simulink model "aeroplt2"  (Simulink 5.0)
settings: Solver=ode1  StartTime=0.0  StopTime=t_in(end)  FixedStep=.02  RelTol=1e-3
values from neighbouring files (symbols this model uses):
  b = 124.524    [gp.m]    (also in trim_541.mat)
  Cbar = 16.64    [gp.m]    (also in trim_541.mat)
  CG = 0.25    [gp.m]    (also in trim_541.mat)
  cs = 1100    [gp.m]    (also in trim_541.mat = 1097.09545231)
  EAS = 210    [gp.m]    (also in trim_541.mat = 209.982128693)
  QBAR = 150    [gp.m]    (also in trim_541.mat = 149.275292764)
  RunwayAlt = 9    [gp.m]    (also in trim_541.mat)
  S = 1951    [gp.m]    (also in trim_541.mat)
  splr_vec = 0:splr_step:10    [gp.m]    (also in gp.mat = [0 2 4 6 8 10])
  StatesInp = [380.111621264 0 35.7647907785 0 -1.82640716025e-05 0 5000 0.698131700798 -1.29154364648 0 0.0938140386005 0 ... (15 elements, 15x1)]    [trim_541.mat]
  weight = 185000    [gp.m]    (also in trim_541.mat)
libraries: simulink x4
settings Model: Creator=wtb  LastModifiedBy=Gpapageo  ExtModeAutoUpdateStatusClock=off  BooleanDataType=off

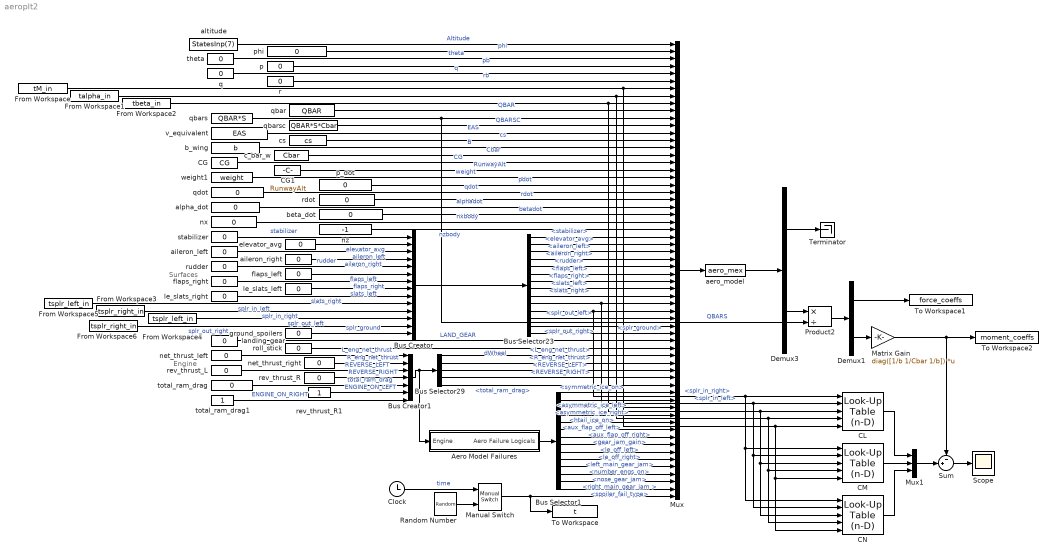
== system aeroplt2 ==
  note: Surfaces
  note: Engine
  " aileron_right" : Constant  Value=0
  Aero Model Failures : Subsystem
  Bus Creator : BusCreator  Inputs=14
  Bus Creator1 : BusCreator  Inputs=7
  Bus Selector1 : BusSelector  OutputSignals=symmetric_ice_on,asymmetric_ice_left,asymmetric_ice_right,htail_ice_on,aux_flap_off_left,aux_flap_off_right,gear_jam_gain,le_off_left,le_off_right,left_main_gear_jam,number_engs_on,nose_gear_jam,right_main_gear_jam ,spoiler_fail_type
  Bus Selector23 : BusSelector  OutputSignals=stabilizer,elevator_avg,aileron_left,aileron_right,rudder,flaps_left,flaps_right,slats_left,slats_right,splr_in_left,splr_in_right,splr_out_left,splr_out_right,splr_ground
  Bus Selector29 : BusSelector  OutputSignals=L_eng_net_thrust,R_eng_net_thrust,REVERSE_LEFT,REVERSE_RIGHT,total_ram_drag
  CG : Constant  Value=CG
  CG1 : Constant  Value=RunwayAlt
  CL : simulink/Look-Up Tables/Look-Up Table (n-D)  numDimsPopupSelect=More...  bp1=splr_vec  bp2=splr_vec  bp3=beta_vec  bp4=alpha_vec  bpcell={M_vec}  explicitNumDims=5  searchMode=Binary Search  cacheBpFlag=on  vectorInputFlag=off  tableData=CL_mat  interpMethod=Linear  extrapMethod=Linear  rangeErrorMode=None
  CM : simulink/Look-Up Tables/Look-Up Table (n-D)  numDimsPopupSelect=More...  bp1=splr_vec  bp2=splr_vec  bp3=beta_vec  bp4=alpha_vec  bpcell={M_vec}  explicitNumDims=5  searchMode=Binary Search  cacheBpFlag=on  vectorInputFlag=off  tableData=CM_mat  interpMethod=Linear  extrapMethod=Linear  rangeErrorMode=None
  CN : simulink/Look-Up Tables/Look-Up Table (n-D)  numDimsPopupSelect=More...  bp1=splr_vec  bp2=splr_vec  bp3=beta_vec  bp4=alpha_vec  bpcell={M_vec}  explicitNumDims=5  searchMode=Binary Search  cacheBpFlag=on  vectorInputFlag=off  tableData=CN_mat  interpMethod=Linear  extrapMethod=Linear  rangeErrorMode=None
  Clock : Clock
      settings: Decimation=10
  Demux1 : Demux  Outputs=[3 3]
  Demux3 : Demux  Outputs=[7 6]
  From Workspace : FromWorkspace  VariableName=tM_in  SampleTime=.02
  From Workspace1 : FromWorkspace  VariableName=talpha_in  SampleTime=.02
  From Workspace2 : FromWorkspace  VariableName=tbeta_in  SampleTime=.02
  From Workspace3 : FromWorkspace  VariableName=tsplr_right_in  SampleTime=.02
  From Workspace4 : FromWorkspace  VariableName=tsplr_left_in  SampleTime=.02
  From Workspace5 : FromWorkspace  VariableName=tsplr_left_in  SampleTime=.02
  From Workspace6 : FromWorkspace  VariableName=tsplr_right_in  SampleTime=.02
  Manual Switch : simulink/Signal Routing/Manual Switch  sw=1  action=0
  Matrix Gain : Gain  Gain=diag([1/b 1/Cbar 1/b])  Multiplication=Matrix(K*u)  SaturateOnIntegerOverflow=on
  Mux : Mux  Inputs=62
  Mux1 : Mux  Inputs=3
  Product2 : Product  Inputs=*/  SaturateOnIntegerOverflow=on
  Random Number : RandomNumber  SampleTime=0
  Scope : Scope
      settings: YMin=-3.5e-018  YMax=3.5e-018
  Sum : Sum  Inputs=-+|  SaturateOnIntegerOverflow=on
  Terminator : Terminator
  To Workspace : ToWorkspace  VariableName=t  SampleTime=.02  SaveFormat=Array
  To Workspace1 : ToWorkspace  VariableName=force_coeffs  SampleTime=-1  SaveFormat=Array
  To Workspace2 : ToWorkspace  VariableName=moment_coeffs  SampleTime=-1  SaveFormat=Array
  aero_model : S-Function  FunctionName=aero_mex
  aileron_left : Constant  Value=0
  alpha_dot : Constant  Value=0
  altitude : Constant  Value=StatesInp(7)
  b_wing : Constant  Value=b
  beta_dot : Constant  Value=0
  c_bar_w : Constant  Value=Cbar
  cs : Constant  Value=cs
  elevator_avg : Constant  Value=0
  flaps_left : Constant  Value=0
  flaps_right : Constant  Value=0
  ground_spoilers : Constant  Value=0
  landing_gear : Constant  Value=0
  le_slats_left : Constant  Value=0
  le_slats_right : Constant  Value=0
  net_thrust_left : Constant  Value=0
  net_thrust_right : Constant  Value=0
  nx : Constant  Value=0
  nz : Constant  Value=-1
  p : Constant  Value=0
  p_dot : Constant  Value=0
  phi : Constant  Value=0
  q : Constant  Value=0
  qbar : Constant  Value=QBAR
  qbars : Constant  Value=QBAR*S
  qbarsc : Constant  Value=QBAR*S*Cbar
  qdot : Constant  Value=0
  r : Constant  Value=0
  rdot : Constant  Value=0
  rev_thrust_L : Constant  Value=0
  rev_thrust_R : Constant  Value=0
  rev_thrust_R1 : Constant
  roll_stick : Constant  Value=0
  rudder : Constant  Value=0
  stabilizer : Constant  Value=0
  theta : Constant  Value=0
  total_ram_drag : Constant  Value=0
  total_ram_drag1 : Constant
  v_equivalent : Constant  Value=EAS
  weight1 : Constant  Value=weight
  wires:
  aero_model/1 -> Demux3/1
  altitude/1 -> Mux/1  "Altitude"
  beta_dot/1 -> Mux/24  "betadot"
  phi/1 -> Mux/2  "phi"
  qbar/1 -> Mux/10  "QBAR"
  qbarsc/1 -> Mux/12  "QBARSC"
  v_equivalent/1 -> Mux/13  "EAS"
  cs/1 -> Mux/14  "cs"
  b_wing/1 -> Mux/15  "B"
  c_bar_w/1 -> Mux/16  "Cbar"
  CG/1 -> Mux/17  "CG"
  weight1/1 -> Mux/19  "weight"
  p_dot/1 -> Mux/20  "pdot"
  qdot/1 -> Mux/21  "qdot"
  rdot/1 -> Mux/22  "rdot"
  alpha_dot/1 -> Mux/23  "alphadot"
  nx/1 -> Mux/25  "nxbody"
  nz/1 -> Mux/26  "nzbody"
  stabilizer/1 -> Bus Creator/1  "stabilizer"
  elevator_avg/1 -> Bus Creator/2  "elevator_avg"
  aileron_left/1 -> Bus Creator/3  "aileron_left"
  " aileron_right"/1 -> Bus Creator/4  "aileron_right"
  rudder/1 -> Bus Creator/5  "rudder"
  flaps_left/1 -> Bus Creator/6  "flaps_left"
  flaps_right/1 -> Bus Creator/7  "flaps_right"
  le_slats_left/1 -> Bus Creator/8  "slats_left"
  le_slats_right/1 -> Bus Creator/9  "slats_right"
  From Workspace5/1 -> Bus Creator/10  "splr_in_left"
  From Workspace3/1 -> Bus Creator/11  "splr_in_right"
  From Workspace4/1 -> Bus Creator/12  "splr_out_left"
  ground_spoilers/1 -> Bus Creator/14  "splr_ground"
  landing_gear/1 -> Mux/41  "LAND_GEAR"
  roll_stick/1 -> Mux/42  "dWheel"
  net_thrust_left/1 -> Bus Creator1/1  "L_eng_net_thrust"
  net_thrust_right/1 -> Bus Creator1/2  "R_eng_net_thrust"
  rev_thrust_L/1 -> Bus Creator1/3  "REVERSE_LEFT"
  rev_thrust_R/1 -> Bus Creator1/4  "REVERSE_RIGHT"
  total_ram_drag/1 -> Bus Creator1/5  "total_ram_drag"
  q/1 -> Mux/5  "q"
  p/1 -> Mux/4  "pb"
  r/1 -> Mux/6  "rb"
  qbars/1 -> Mux/11, Product2/2  "QBARS"
  theta/1 -> Mux/3  "theta"
  CG1/1 -> Mux/18  "RunwayAlt"
  Aero Model Failures/1(Aero Failure Logicals) -> Bus Selector1/1
  Bus Creator1/1 -> Bus Selector29/1, Aero Model Failures/1(Engine)
  Bus Selector23/1 -> Mux/27  "<stabilizer>"
  Bus Selector23/2 -> Mux/28  "<elevator_avg>"
  Bus Selector23/3 -> Mux/29  "<aileron_left>"
  Bus Selector23/4 -> Mux/30  "<aileron_right>"
  Mux/1 -> aero_model/1
  Bus Selector23/5 -> Mux/31  "<rudder>"
  Bus Selector23/6 -> Mux/32  "<flaps_left>"
  Bus Selector23/7 -> Mux/33  "<flaps_right>"
  Bus Selector23/8 -> Mux/34  "<slats_left>"
  Bus Selector23/9 -> Mux/35  "<slats_right>"
  Bus Selector23/10 -> Mux/36, CL/2, CM/2, CN/2  "<splr_in_left>"
  Bus Selector23/11 -> Mux/37, CL/1, CM/1, CN/1  "<splr_in_right>"
  Bus Selector23/12 -> Mux/38  "<splr_out_left>"
  Bus Selector23/13 -> Mux/39  "<splr_out_right>"
  Bus Selector23/14 -> Mux/40  "<splr_ground>"
  Bus Selector29/1 -> Mux/43  "<L_eng_net_thrust>"
  Bus Selector29/2 -> Mux/44  "<R_eng_net_thrust>"
  Bus Selector29/3 -> Mux/45  "<REVERSE_LEFT>"
  Bus Selector29/4 -> Mux/46  "<REVERSE_RIGHT>"
  Bus Selector29/5 -> Mux/47  "<total_ram_drag>"
  Bus Selector1/1 -> Mux/48  "<symmetric_ice_on>"
  Bus Selector1/2 -> Mux/49  "<asymmetric_ice_left>"
  Bus Selector1/3 -> Mux/50  "<asymmetric_ice_right>"
  Bus Selector1/4 -> Mux/51  "<htail_ice_on>"
  Bus Selector1/5 -> Mux/52  "<aux_flap_off_left>"
  Bus Selector1/6 -> Mux/53  "<aux_flap_off_right>"
  Bus Selector1/7 -> Mux/54  "<gear_jam_gain>"
  Bus Selector1/8 -> Mux/55  "<le_off_left>"
  Bus Selector1/9 -> Mux/56  "<le_off_right>"
  Bus Selector1/10 -> Mux/57  "<left_main_gear_jam>"
  Bus Selector1/11 -> Mux/58  "<number_engs_on>"
  Bus Selector1/12 -> Mux/59  "<nose_gear_jam>"
  Bus Selector1/13 -> Mux/60  "<right_main_gear_jam >"
  Bus Selector1/14 -> Mux/61  "<spoiler_fail_type>"
  rev_thrust_R1/1 -> Bus Creator1/6  "ENGINE_ON_LEFT"
  total_ram_drag1/1 -> Bus Creator1/7  "ENGINE_ON_RIGHT"
  Manual Switch/1 -> Mux/62, To Workspace/1
  Clock/1 -> Manual Switch/1  "time"
  Random Number/1 -> Manual Switch/2
  From Workspace/1 -> Mux/7, CL/5, CM/5, CN/5
  From Workspace1/1 -> Mux/8, CL/4, CM/4, CN/4
  From Workspace2/1 -> Mux/9, CL/3, CM/3, CN/3
  From Workspace6/1 -> Bus Creator/13  "splr_out_right"
  Bus Creator/1 -> Bus Selector23/1
  Product2/1 -> Demux1/1
  Demux1/2 -> Matrix Gain/1
  Demux3/1 -> Terminator/1
  Demux3/2 -> Product2/1
  Matrix Gain/1 -> To Workspace2/1, Sum/1
  Demux1/1 -> To Workspace1/1
  Sum/1 -> Scope/1
  CM/1 -> Mux1/2
  CL/1 -> Mux1/1
  CN/1 -> Mux1/3
  Mux1/1 -> Sum/2

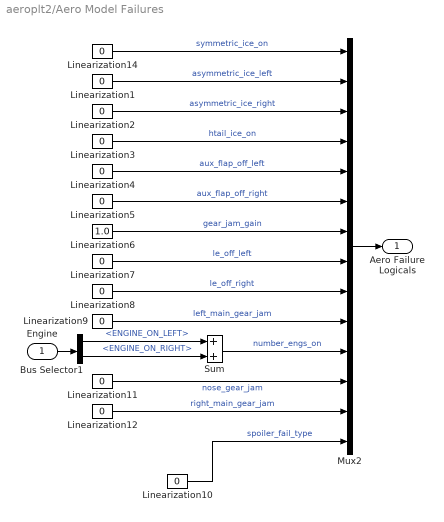
== system aeroplt2/Aero Model Failures ==
  Engine : Inport
  Bus Selector1 : BusSelector  OutputSignals=ENGINE_ON_LEFT,ENGINE_ON_RIGHT
  Linearization{1..5,7..12,14} (12 alike) : Constant  Value=0
  Linearization6 : Constant  Value=1.0
  Mux2 : Mux  Inputs=14
  Sum : Sum  SaturateOnIntegerOverflow=on  InputSameDT=on
  Aero Failure Logicals : Outport
  wires:
  Mux2/1 -> Aero Failure Logicals/1
  Linearization4/1 -> Mux2/5  "aux_flap_off_left"
  Linearization6/1 -> Mux2/7  "gear_jam_gain"
  Sum/1 -> Mux2/11  "number_engs_on"
  Linearization11/1 -> Mux2/12  "nose_gear_jam"
  Linearization14/1 -> Mux2/1  "symmetric_ice_on"
  Linearization1/1 -> Mux2/2  "asymmetric_ice_left"
  Linearization2/1 -> Mux2/3  "asymmetric_ice_right"
  Linearization3/1 -> Mux2/4  "htail_ice_on"
  Linearization5/1 -> Mux2/6  "aux_flap_off_right"
  Linearization7/1 -> Mux2/8  "le_off_left"
  Linearization8/1 -> Mux2/9  "le_off_right"
  Linearization9/1 -> Mux2/10  "left_main_gear_jam"
  Linearization12/1 -> Mux2/13  "right_main_gear_jam"
  Engine/1 -> Bus Selector1/1
  Bus Selector1/1 -> Sum/1  "<ENGINE_ON_LEFT>"
  Bus Selector1/2 -> Sum/2  "<ENGINE_ON_RIGHT>"
  Linearization10/1 -> Mux2/14  "spoiler_fail_type"
